simulink model "Impdc_CNTRL_v1"  (R2021a)
settings: Solver=ode4  StartTime=0.0  StopTime=max(t2)  FixedStep=dt  RelTol=1e-3
values from neighbouring files (symbols this model uses):
  D = [b1*dthd(1,i);b2*dthd(2,i)]    [VILC.m]
  dt = 1/100    (= 0.01)    [VILC.m]
  F = 1    [VILC.m]
  K = Ka+Kp    [VILC.m]
  th1i = q1(1) +  0*rand/100    [VILC.m]
  th2i = q2(1) +  0*rand/100    [VILC.m]
settings Model: Creator=shail  LastModifiedBy=shail
settings SolverCC: AlgebraicLoopSolver=TrustRegion
settings DebuggingCC: SFMachineParentedDataDiag=warning

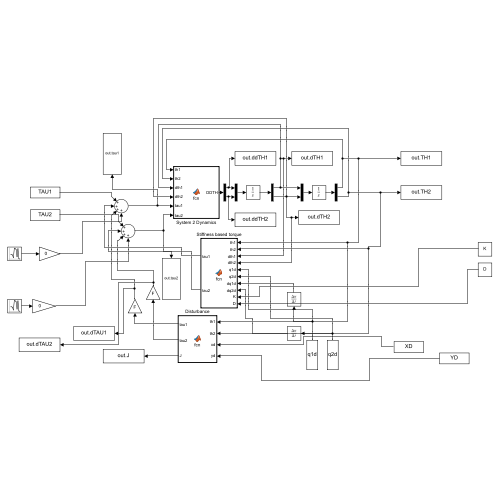
[thumbnail: Simulink's stored preview of the top-level diagram]
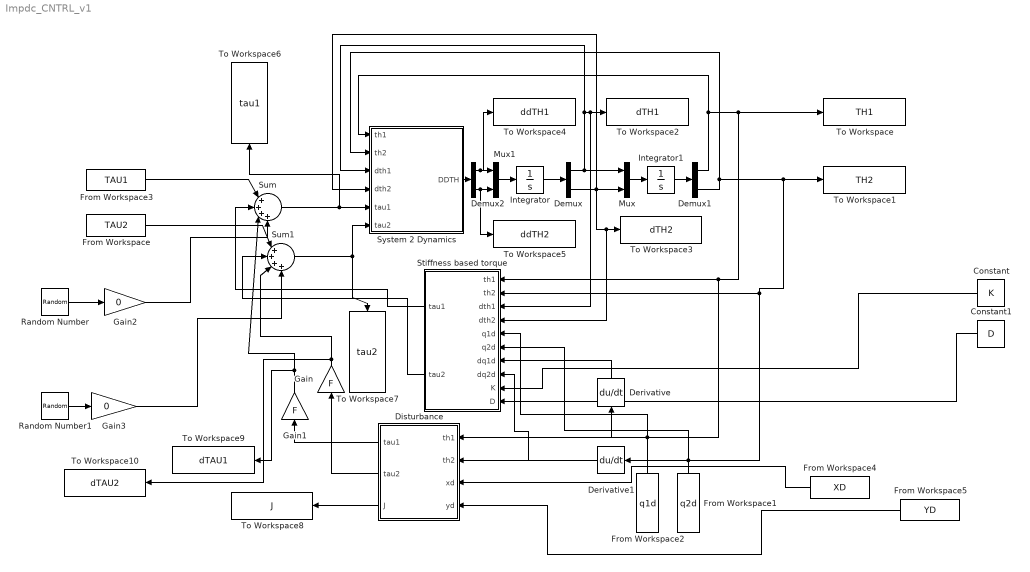
== system Impdc_CNTRL_v1 ==
  Constant : Constant  Value=K
  Constant1 : Constant  Value=D
  Demux : Demux  Outputs=2
  Demux1 : Demux  Outputs=2
  Demux2 : Demux  Outputs=2
  Derivative : Derivative
  Derivative1 : Derivative
  Disturbance : MATLAB Function  TreatAsAtomicUnit=on
  From Workspace : FromWorkspace  VariableName=TAU2
  From Workspace1 : FromWorkspace  VariableName=q2d
  From Workspace2 : FromWorkspace  VariableName=q1d
  From Workspace3 : FromWorkspace  VariableName=TAU1
  From Workspace4 : FromWorkspace  VariableName=XD
  From Workspace5 : FromWorkspace  VariableName=YD
  Gain : Gain  Gain=F
  Gain1 : Gain  Gain=F
  Gain2 : Gain  Gain=0
  Gain3 : Gain  Gain=0
  Integrator : Integrator  InitialCondition=[0;0]
  Integrator1 : Integrator  InitialCondition=[th1i;th2i]
  Mux : Mux  Inputs=2
  Mux1 : Mux  Inputs=2
  Random Number : RandomNumber  Variance=2  SampleTime=dt
  Random Number1 : RandomNumber  Variance=2  SampleTime=dt
  Stiffness based torque : MATLAB Function  TreatAsAtomicUnit=on
  Sum : Sum  Inputs=|++++
  Sum1 : Sum  Inputs=|++++
  System 2 Dynamics : MATLAB Function  TreatAsAtomicUnit=on
  To Workspace : ToWorkspace  VariableName=TH1  SaveFormat=Timeseries  SampleTime=-1
  To Workspace1 : ToWorkspace  VariableName=TH2  SaveFormat=Timeseries  SampleTime=-1
  To Workspace10 : ToWorkspace  VariableName=dTAU2  SaveFormat=Timeseries  SampleTime=-1
  To Workspace2 : ToWorkspace  VariableName=dTH1  SaveFormat=Timeseries  SampleTime=-1
  To Workspace3 : ToWorkspace  VariableName=dTH2  SaveFormat=Timeseries  SampleTime=-1
  To Workspace4 : ToWorkspace  VariableName=ddTH1  SaveFormat=Timeseries  SampleTime=-1
  To Workspace5 : ToWorkspace  VariableName=ddTH2  SaveFormat=Timeseries  SampleTime=-1
  To Workspace6 : ToWorkspace  VariableName=tau1  SaveFormat=Timeseries  SampleTime=-1
  To Workspace7 : ToWorkspace  VariableName=tau2  SaveFormat=Timeseries  SampleTime=-1
  To Workspace8 : ToWorkspace  VariableName=J  SaveFormat=Timeseries  SampleTime=-1
  To Workspace9 : ToWorkspace  VariableName=dTAU1  SaveFormat=Timeseries  SampleTime=-1
  wires:
  Integrator/1 -> Demux/1
  Mux/1 -> Integrator1/1
  Demux/1 -> Stiffness based torque/3(dth1), To Workspace2/1, System 2 Dynamics/3(dth1), Mux/1
  Integrator1/1 -> Demux1/1
  Demux1/1 -> Disturbance/1(th1), Stiffness based torque/1(th1), To Workspace/1, System 2 Dynamics/1(th1)
  Demux/2 -> Stiffness based torque/4(dth2), To Workspace3/1, Mux/2, System 2 Dynamics/4(dth2)
  Demux1/2 -> System 2 Dynamics/2(th2), Disturbance/2(th2), Stiffness based torque/2(th2), To Workspace1/1
  From Workspace2/1 -> Stiffness based torque/5(q1d), Derivative/1
  From Workspace3/1 -> Sum/1
  From Workspace/1 -> Sum1/1
  Stiffness based torque/1(tau1) -> Sum/2
  Stiffness based torque/2(tau2) -> Sum1/2
  System 2 Dynamics/1(DDTH) -> Demux2/1
  Demux2/1 -> To Workspace4/1, Mux1/1
  Demux2/2 -> To Workspace5/1, Mux1/2
  Mux1/1 -> Integrator/1
  From Workspace1/1 -> Stiffness based torque/6(q2d), Derivative1/1
  Derivative/1 -> Stiffness based torque/7(dq1d)
  Derivative1/1 -> Stiffness based torque/8(dq2d)
  From Workspace4/1 -> Disturbance/3(xd)
  From Workspace5/1 -> Disturbance/4(yd)
  Disturbance/1(tau1) -> Gain1/1
  Disturbance/2(tau2) -> Gain/1
  Gain/1 -> Sum1/3, To Workspace10/1
  Gain1/1 -> To Workspace9/1, Sum/3
  Random Number/1 -> Gain2/1
  Gain2/1 -> Sum/4
  Random Number1/1 -> Gain3/1
  Gain3/1 -> Sum1/4
  Constant/1 -> Stiffness based torque/9(K)
  Constant1/1 -> Stiffness based torque/10(D)
  Sum/1 -> System 2 Dynamics/5(tau1), To Workspace6/1
  Sum1/1 -> System 2 Dynamics/6(tau2), To Workspace7/1
  Disturbance/3(J) -> To Workspace8/1

== matlab function Impdc_CNTRL_v1/Stiffness based torque ==
  data: tau1 output; th1 input; tau2 output; th2 input; dth1 input; dth2 input; q1d input; q2d input; dq1d input; dq2d input; K input; D input
function [tau1,tau2] = fcn(th1,th2,dth1,dth2,q1d,q2d,dq1d,dq2d,K,D)
q1e=q1d-th1;
q2e=q2d-th2;
qe=[q1e;q2e];
dq1e=dq1d-dth1;
dq2e=dq2d-dth2;
dqe=[dq1e;dq2e];
T=K*(qe)+D*dqe;

tau1=1*T(1);
tau2=1*T(2);

== matlab function Impdc_CNTRL_v1/System 2 Dynamics ==
  data: th1 input; DDTH output; th2 input; dth1 input; dth2 input; tau1 input; tau2 input
function DDTH = fcn(th1,th2,dth1,dth2,tau1,tau2)

%%%%%%%%%%%%%%%%%%%%%%%
m1 = 1 ;
m2 = 1 ; g = 0 ;
l1 = 1 ; lc1 = l1/2 ;
l2 = 1 ; lc2 = l2/2 ;
I1 = 1/12 ; I2 = 1/12 ;
b1=0.5;
b2=0.5;


%%
M = [m1*lc1^2 + m2*(l1^2+lc2^2+2*l1*lc2^2+2*l1*lc2*cos(th2)) + I1 + I2, m2*(lc2^2 + l1*lc2*cos(th2)) + I2;
    m2*(lc2^2 + l1*lc2*cos(th2)) + I2, m2*lc2^2 + I2] ;
C = [-m2*l1*lc2*sin(th2)*dth2, -m2*l1*lc2*sin(th2)*dth2 - m2*l1*lc2*sin(th2)*dth1;
    m2*l1*lc2*sin(th2)*dth1, 0] ;
G = [(m1*lc1 + m2*l1)*g*cos(th1) + m2*lc2*g*cos(th1 + th2);
    m2*lc2*g*cos(th1+th2)] ;
D=[b1*dth1;b2*dth2];

% ddth_b(:,i+1) = inv(M)*(Tau(:,i) - C*dth_b(:,i) - G)

tau=[tau1;tau2];
dth=[dth1;dth2];

DDTH=inv(M)*(tau-D-C*dth);




%%%%%%%%%%%%%%%%%%%%%%%%




% m1=1;
% m2=1;
% b1=0.5;
% b2=0.5;
% L1=1;
% L2=1;
% 
% dth=[dth1;dth2];
% tau=[tau1;tau2];
% M11=(4*L1^2*m1)/3 + L1^2*m2 + L2^2*m2 + 2*L1*L2*m2*cos(th2);
% M12=m2*L2^2 + L1*m2*cos(th2)*L2;
% M21=m2*L2^2 + L1*m2*cos(th2)*L2;
% M22=(4*L2^2*m2)/3;
% 
% M=[M11 M12;M21 M22];
% 
% C11=-2*L1*L2*m2*sin(th2)*dth2;
% C12=- L1*L2*m2*sin(th2) - 2*L1*L2*m2*sin(th2)*dth1;
% C21=L1*L2*m2*sin(th2);
% C22=0;
% C=[C11 C12;C21 C22];
% 
% D=[b1*dth1;b2*dth2];
% DDTH=inv(M)*(tau-D-C*dth);

% M11=((((m1/3) + m2)*l1^2) +((m2/3)*l2^2) + (m2*l1*l2*cos(th2)));
% M12=(m2*(((l2^2)/3) + (0.5*l1*l2*cos(th2))));
% M21=M12;
% M22=((1/3)*m2*l2*l2);
%
% M=[M11 M12;M21 M22];
%
% H1 =((-m2*l1*l2*sin(th2)*dth1*dth2) - (0.5*m2*l1*l2*sin(th2)*dth2*dth2));
% H2 = (0.5 * m2* l1*l2*sin(th2)*dth1*dth1);
% G1=( ((((0.5*m1) + m2)*l1*cos(th1)) + (0.5*m2*l2*cos(th1+th2)))*g);
% G2=0.5*m2*l2*cos(th1+th2)*g;

== matlab function Impdc_CNTRL_v1/Disturbance ==
  data: tau1 output; th1 input; tau2 output; th2 input; xd input; yd input; J output
function [tau1,tau2,J] = fcn(th1,th2,xd,yd)
l1=1;
l2=1;
xc=l1*cos(th1)+l2*cos(th1+th2);
yc=l1*sin(th1)+l2*sin(th1+th2);
J=[-l1*sin(th1)-l2*sin(th2),-l2*sin(th1+th2);l1*cos(th1)+l2*cos(th1+th2),l2*cos(th1+th2)];
k1=-5;%20
k2=-5;%20
K=[k1 0;0 k2];
th=0;
R=[cos(th) -sin(th);sin(th) cos(th)];
Xe=[xd-xc;yd-yc];
T=J'*K*R*Xe;
tau1=T(1);
tau2=T(2);
